simulink model "vrlights"  (Simulink 7.4)
settings: Solver=ode45  StartTime=0.0  StopTime=Inf  RelTol=1e-3
libraries: vrlib x1
Description:
  | Variable Lighting
  | 
  | vrlights is an example with light sources. In the scene there are Sun (modeled as
  | DirectionalLight) and Lamp (modeled as PointLight) moved around from the Simulink(R)
  | model, creating the illusion of changes between day and night terrain illumination. In the
  | associated VRML file, several viewpoints are defined that allow you to observe gradual
  | changes in light from various perspectives.
  | 
  | While the effect of moving light sources on the terrain is directly visible, the VRML world
  | background doesn't automatically reflect the current light sources status. Background
  | color needs to be specifically changed depending on the Sun position. Here it is done
  | using a VRMLScript. For details please view the associated VRML file vrlights.wrl in a text
  | editor.
  | 
  | This example can be used for training user navigation and testing the use of navigation
  | zones in various navigation modes.
settings Model: Creator=Straka  LastModifiedBy=Houska  CovMetricSettings=d  ExtModeTrigMode=oneshot  ExtModeArmWhenConnect=off
settings DataIOCC: LimitDataPoints=off  SaveOutput=off  SaveTime=off  SignalLoggingName=logsOut
settings OptimizationCC: BlockReduction=off  BooleanDataType=off  InlineInvariantSignals=on  InitFltsAndDblsToZero=on
settings DebuggingCC: CheckExecutionContextPreStartOutputMsg=on  CheckExecutionContextRuntimeOutputMsg=on  SignalResolutionControl=TryResolveAllWithWarning  SolverPrmCheckMsg=none  MultiTaskDSMMsg=warning  MultiTaskCondExecSysMsg=none  StrictBusMsg=None
settings HardwareCC: TargetUnknown=on
settings ModelReferenceCC: UpdateModelReferenceTargets=IfOutOfDate
settings SFSimCC: SimGenerateEmlReport=off
settings RTWCC: IncludeERTFirstTime=on
settings GRTTargetCC: TargetFcnLib=ansi_tfl_tmw.mat

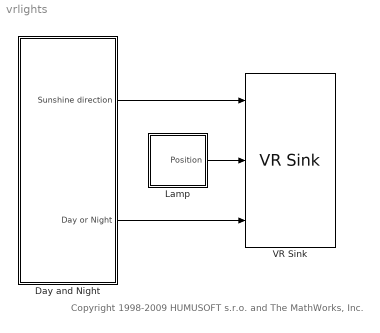
== system vrlights ==
  note: Copyright 1998-2009 HUMUSOFT s.r.o. and The MathWorks, Inc.
  Day and Night : Subsystem
  Lamp : Subsystem
  VR Sink : vrlib/VR Sink  InstantiateOnLoad=on  SampleTime=0.1  ViewEnable=on  RemoteChange=off  RemoteView=off  FieldsWritten=Sun.direction.3.1.double#Lamp.location.3.1.double#Lamp.on.1.1.logical  WorldFileName=vrlights.wrl  AutoView=on  VideoDimensions=[]  FigureProperties="{'Position', 'Name', 'Viewpoint', 'CameraBound', 'CameraDirection', 'CameraPosition', 'CameraUpVector', 'ZoomFactor', 'Antialiasing', 'Headlight', 'Lighting', 'NavPanel', 'StatusBar', 'ToolBar', 'Textures', 'Transparency', 'Wireframe', 'NavZones', 'NavMode', 'NavSpeed', 'Record2DCompressMethod', 'Record2DCompressQuality', 'Record2D', 'Record2DFileName', 'Record2DFPS'; [5.0000000000000000e+000  9.2000000000000000e+001  5.7600000000000000e+002  3.8000000000000000e+002], 'Variable Lighting Example', 'Mount St. Barbara', 'on', [0.0000000000000000e+000  0.0000000000000000e+000 -1.0000000000000000e+000], [0.0000000000000000e+000  0.0000000000000000e+000  0.0000000000000000e+000], [0.0000000000000000e+000  1.0000000000000000e+000  0.0000000000000000e+000], [1.0000000000000000e+000], 'off', 'off', 'on', 'halfbar', 'on', 'on', 'on', 'on', 'off', 'off', 'fly', 'normal', 'auto', [7.5000000000000000e+001], 'off', '%f_anim_%n.avi', [1.5000000000000000e+001]}"
  wires:
  Lamp/1(Position) -> VR Sink/2
  Day and Night/2(Day or Night) -> VR Sink/3
  Day and Night/1(Sunshine direction) -> VR Sink/1

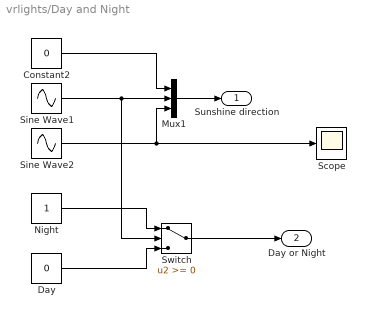
== system vrlights/Day and Night ==
  Constant2 : Constant  Value=0  OutDataType=sfix(16)  OutScaling=2^0
  Day : Constant  Value=0  OutDataType=sfix(16)  OutScaling=2^0
  Mux1 : Mux  Inputs=3
  Night : Constant  OutDataType=sfix(16)  OutScaling=2^0
  Scope : Scope
  Sine Wave1 : Sin  Amplitude=1  Bias=0  Frequency=0.03  Phase=-1.57  Samples=10  SampleTime=0  Offset=0
  Sine Wave2 : Sin  Amplitude=1  Bias=0  Frequency=0.03  Phase=0  Samples=10  SampleTime=0  Offset=0
  Switch : Switch  OutDataType=sfix(16)  OutScaling=2^0  InputSameDT=on
  Sunshine direction : Outport  OutDataType=sfix(16)  OutScaling=2^0
  Day or Night : Outport  Port=2  OutDataType=sfix(16)  OutScaling=2^0
  wires:
  Constant2/1 -> Mux1/1
  Mux1/1 -> Sunshine direction/1
  Night/1 -> Switch/1
  Day/1 -> Switch/3
  Sine Wave1/1 -> Mux1/2, Switch/2
  Sine Wave2/1 -> Mux1/3, Scope/1
  Switch/1 -> Day or Night/1

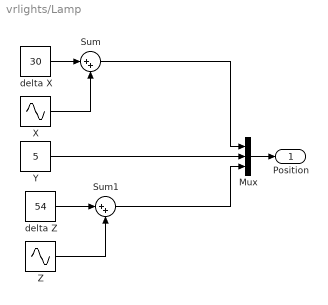
== system vrlights/Lamp ==
  Mux : Mux  Inputs=3
  Sum : Sum  Inputs=|++  OutDataType=sfix(16)  OutScaling=2^0  SaturateOnIntegerOverflow=on  InputSameDT=on  OutDataTypeStr=Inherit: Same as first input
  Sum1 : Sum  Inputs=|++  OutDataType=sfix(16)  OutScaling=2^0  SaturateOnIntegerOverflow=on  InputSameDT=on  OutDataTypeStr=Inherit: Same as first input
  X : Sin  Amplitude=20  Bias=0  Frequency=0.065  Phase=0  Samples=10  SampleTime=0  Offset=0
  Y : Constant  Value=5  OutDataType=sfix(16)  OutScaling=2^0
  Z : Sin  Amplitude=24  Bias=0  Frequency=0.05  Phase=0  Samples=10  SampleTime=0  Offset=0
  delta X : Constant  Value=30  OutDataType=sfix(16)  OutScaling=2^0
  delta Z : Constant  Value=54  OutDataType=sfix(16)  OutScaling=2^0
  Position : Outport  OutDataType=sfix(16)  OutScaling=2^0
  wires:
  delta X/1 -> Sum/1
  Y/1 -> Mux/2
  delta Z/1 -> Sum1/1
  Mux/1 -> Position/1
  Sum1/1 -> Mux/3
  Sum/1 -> Mux/1
  Z/1 -> Sum1/2
  X/1 -> Sum/2
